simulink library "sixDoFKinematics_ul"  (R2018b)
settings: Solver=VariableStepAuto  StartTime=0.0  StopTime=10.0  RelTol=1e-3
undefined symbols (not defined in the file): initAngRates, initEulAngs, initPos, initVel, Jinv
libraries: vrlib x2
settings Model: Creator=mcobb  LastModifiedBy=mcobb

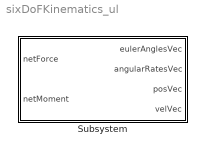
== system sixDoFKinematics_ul ==
  Subsystem : Subsystem  mask{J=eye(3), m=1, Parameter3=0, Parameter4=0}
      mask prompts: J "Inertia matrix"; m "Mass"; Parameter3 "Initial Euler Angles"; Parameter4 "Initial Angular Rates"
      mask init:
      | sixDoFKinematics_init

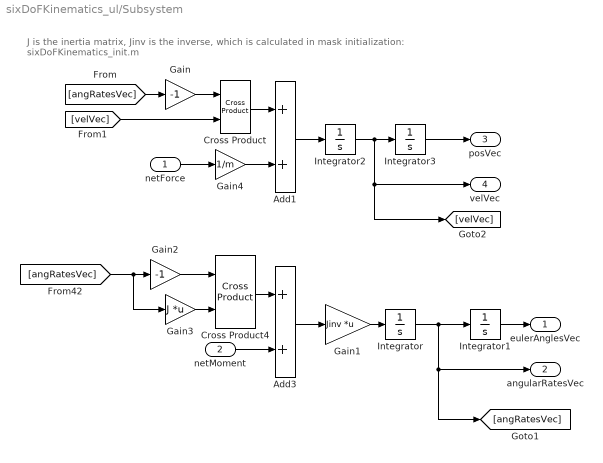
== system sixDoFKinematics_ul/Subsystem ==
  note: J is the inertia matrix, Jinv is the inverse, which is calculated in mask initialization: sixDoFKinematics_init.m
  netForce : Inport
  netMoment : Inport  Port=2
  Add1 : Sum
  Add3 : Sum
  Cross Product : vrlib/Utilities/Cross Product
      settings: SourceProductBaseCode=VR
  Cross Product4 : vrlib/Utilities/Cross Product
      settings: SourceProductBaseCode=VR
  Gain : Gain  Gain=-1
  Gain1 : Gain  Gain=Jinv  Multiplication=Matrix(K*u)
  Gain2 : Gain  Gain=-1
  Gain3 : Gain  Gain=J  Multiplication=Matrix(K*u)
  Gain4 : Gain  Gain=1/m
  Integrator : Integrator  InitialCondition=initAngRates
  Integrator1 : Integrator  InitialCondition=initEulAngs
  Integrator2 : Integrator  InitialCondition=initVel
  Integrator3 : Integrator  InitialCondition=initPos
  eulerAnglesVec : Outport
  angularRatesVec : Outport  Port=2
  posVec : Outport  Port=3
  velVec : Outport  Port=4
  wires:
  netMoment/1 -> Add3/2
  Gain2/1 -> Cross Product4/1
  Gain3/1 -> Cross Product4/2
  Integrator/1 -> angularRatesVec/1, [angRatesVec], Integrator1/1
  [angRatesVec] -> Gain3/1, Gain2/1
  Add3/1 -> Gain1/1
  Integrator1/1 -> eulerAnglesVec/1
  Gain1/1 -> Integrator/1
  Cross Product4/1 -> Add3/1
  [angRatesVec] -> Gain/1
  Gain/1 -> Cross Product/1
  [velVec] -> Cross Product/2
  Cross Product/1 -> Add1/1
  Gain4/1 -> Add1/2
  netForce/1 -> Gain4/1
  Add1/1 -> Integrator2/1
  Integrator3/1 -> posVec/1
  Integrator2/1 -> [velVec], velVec/1, Integrator3/1
